simulink model "Problem6_FIR_filter"  (R2020b)
settings: Solver=FixedStepAuto  StartTime=0.0  StopTime=50  FixedStep=0.001  RelTol=1e-3
settings Model: Creator=baner  LastModifiedBy=baner

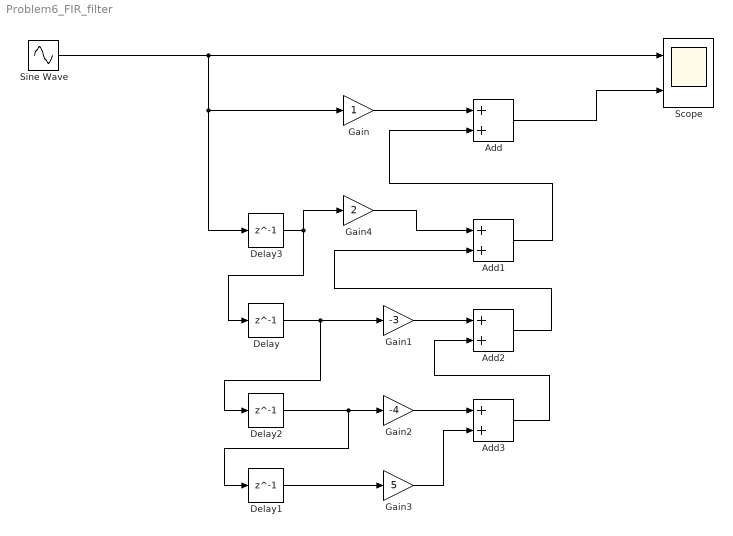
== system Problem6_FIR_filter ==
  Add{,1..3} (4 alike) : Sum
  Delay{,1..3} (4 alike) : Delay  DelayLength=1
  Gain : Gain
  Gain1 : Gain  Gain=-3
  Gain2 : Gain  Gain=-4
  Gain3 : Gain  Gain=5
  Gain4 : Gain  Gain=2
  Scope : Scope  NumInputPorts=2
  Sine Wave : Sin  Frequency=10  SampleTime=0
  wires:
  Sine Wave/1 -> Delay3/1, Gain/1, Scope/1
  Delay3/1 -> Delay/1, Gain4/1
  Delay/1 -> Delay2/1, Gain1/1
  Delay1/1 -> Gain3/1
  Delay2/1 -> Delay1/1, Gain2/1
  Add1/1 -> Add/2
  Add2/1 -> Add1/2
  Add3/1 -> Add2/2
  Add/1 -> Scope/2
  Gain/1 -> Add/1
  Gain4/1 -> Add1/1
  Gain1/1 -> Add2/1
  Gain2/1 -> Add3/1
  Gain3/1 -> Add3/2
